simulink model "Exp_07_02_01"  (R2012b)
settings: Solver=ode3  StartTime=0.0  StopTime=2.0  FixedStep=0.0000001  RelTol=1e-3
libraries: dsparch4 x1
settings Model: Creator=Abraham Xiao  LastModifiedBy=Abraham Xiao
settings RTWCC: GenerateReport=on  LaunchReport=on
settings CodeAppCC: ForceParamTrailComments=on  MATLABSourceComments=on

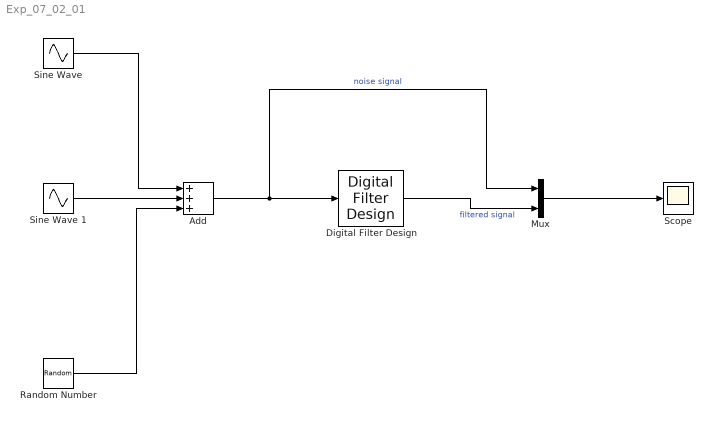
== system Exp_07_02_01 ==
  Add : Sum  Inputs=+++
  Digital Filter Design : dsparch4/Digital Filter Design  mwdsp_browser_bugfix_var=off
  Mux : Mux  Inputs=2
  Random Number : RandomNumber  Variance=0.04  SampleTime=1/1000
  Scope : Scope
      settings: ShowLegends=on  YMin=-3  YMax=3
  "Sine Wave " : Sin  Frequency=10 * 2 * pi  SampleTime=1/1000
  Sine Wave 1 : Sin  Frequency=100 * 2 * pi  SampleTime=1/1000
  wires:
  Sine Wave 1/1 -> Add/2
  "Sine Wave "/1 -> Add/1
  Random Number/1 -> Add/3
  Add/1 -> Mux/1, Digital Filter Design/1  "noise signal"
  Digital Filter Design/1 -> Mux/2  "filtered signal"
  Mux/1 -> Scope/1
